simulink model "problem_6_case1"  (R2018a)
settings: Solver=ode1  StartTime=0.0  StopTime=4  FixedStep=0.0005  RelTol=1e-3
settings Model: Creator=chenxiaocong  LastModifiedBy=LvHonghao
settings CodeAppCC: StateflowObjectComments=on

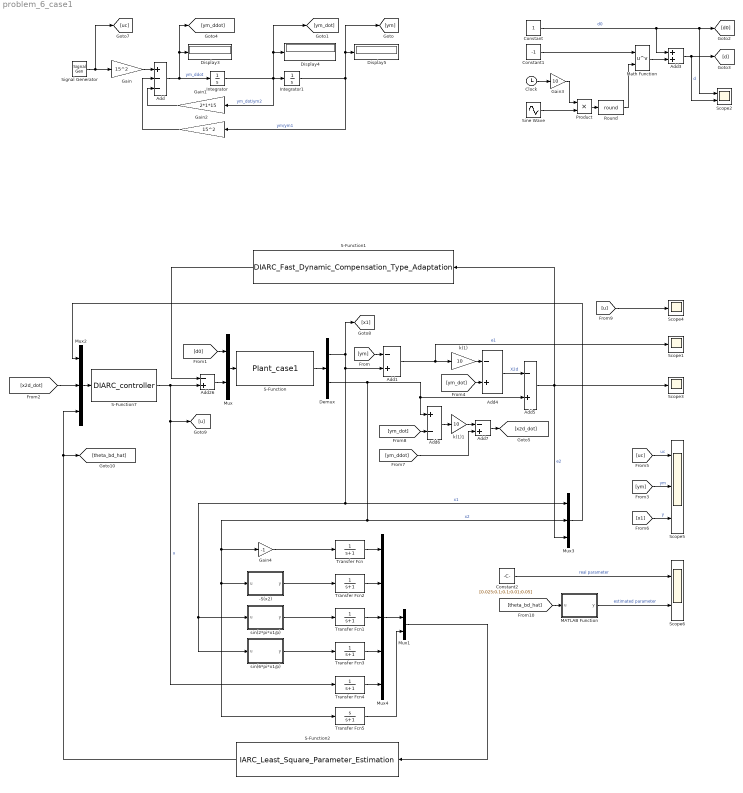
== system problem_6_case1 ==
  -S(x2) : MATLAB Function  TreatAsAtomicUnit=on
  Add : Sum  Inputs=+--
  Add{1,4..5,7,26} (5 alike) : Sum  Inputs=-+
  Add3 : Sum
  Add6 : Sum  Inputs=+-
  Clock : Clock
  Constant : Constant
  Constant1 : Constant  Value=-1
  Constant2 : Constant  Value=[0.025;0.1;0.1;0.01;0.05]
  Demux : Demux  Outputs=2
  Display3 : Display
  Display4 : Display
  Display5 : Display
  Gain : Gain  Gain=15^2
  Gain1 : Gain  Gain=2*1*15
  Gain2 : Gain  Gain=15^2
  Gain3 : Gain  Gain=10
  Gain4 : Gain  Gain=-1
  Integrator : Integrator
  Integrator1 : Integrator
  MATLAB Function : MATLAB Function  TreatAsAtomicUnit=on
  Math Function : Math  Operator=pow  SaturateOnIntegerOverflow=on
  Mux : Mux  Inputs=2
  Mux1 : Mux  Inputs=2
  Mux2 : Mux  Inputs=3
  Mux3 : Mux  Inputs=3
  Mux4 : Mux  Inputs=5
  Product : Product
  Round : Rounding  Operator=round
  S-Function : S-Function  FunctionName=Plant_case1  SFunctionDeploymentMode=off  EnableBusSupport=off
  S-Function1 : S-Function  FunctionName=DIARC_Fast_Dynamic_Compensation_Type_Adaptation  SFunctionDeploymentMode=off  EnableBusSupport=off
  S-Function2 : S-Function  FunctionName=IARC_Least_Square_Parameter_Estimation  SFunctionDeploymentMode=off  EnableBusSupport=off
  S-Function7 : S-Function  FunctionName=DIARC_controller  SFunctionDeploymentMode=off  EnableBusSupport=off
  Scope1 : Scope
  Scope2 : Scope  NumInputPorts=2
  Scope3 : Scope
  Scope4 : Scope
  Scope5 : Scope  NumInputPorts=3
  Scope6 : Scope  NumInputPorts=2
  Signal Generator : SignalGenerator  WaveForm=square  Amplitude=0.1  Frequency=1/1.2
  Sine Wave : Sin  Frequency=20  SampleTime=0
  Transfer Fcn{,1..4} (5 alike) : TransferFcn  Denominator=[1 1]
  Transfer Fcn5 : TransferFcn  Numerator=[1 0]  Denominator=[1 1]
  k(1) : Gain  Gain=10
  k(1)1 : Gain  Gain=10
  sin(2*pi*x1/p) : MATLAB Function  TreatAsAtomicUnit=on
  sin(6*pi*x1/p) : MATLAB Function  TreatAsAtomicUnit=on
  wires:
  Demux/2 -> Mux3/2, Transfer Fcn5/1, -S(x2)/1(u), Gain4/1, Add5/2, Add6/1  "x2"
  Add1/1 -> k(1)/1, Scope1/1  "e1"
  Gain2/1 -> Add/2
  Integrator1/1 -> Gain2/1, [ym], Display5/1  "ym/ym1"
  [ym_dot] -> Add6/2
  Add6/1 -> k(1)1/1
  [ym_dot] -> Add4/2
  Add4/1 -> Add5/1  "X2d"
  S-Function/1 -> Demux/1
  [d0] -> Mux/1
  Mux/1 -> S-Function/1
  Add3/1 -> [d], Scope2/2  "d"
  Constant/1 -> [d0], Scope2/1, Add3/1  "d0"
  k(1)/1 -> Add4/1
  k(1)1/1 -> Add7/1
  Add5/1 -> S-Function1/1, Mux3/3, Scope3/1  "e2"
  Integrator/1 -> Gain1/1, Integrator1/1, [ym_dot], Display4/1  "ym_dot/ym2"
  Gain1/1 -> Add/3
  Demux/1 -> Mux3/1, sin(6*pi*x1/p)/1(u), sin(2*pi*x1/p)/1(u), Add1/2, [x1]  "x1"
  Math Function/1 -> Add3/2
  Round/1 -> Math Function/2
  S-Function7/1 -> [u], Transfer Fcn4/1, Add26/2  "u"
  [ym] -> Add1/1
  Add/1 -> [ym_ddot], Display3/1, Integrator/1  "ym_ddot"
  [ym_ddot] -> Add7/2
  Gain/1 -> Add/1
  Add7/1 -> [x2d_dot]
  Constant1/1 -> Math Function/1
  Mux2/1 -> S-Function7/1
  [x2d_dot] -> Mux2/2
  [ym] -> Scope5/2  "ym"
  [uc] -> Scope5/1  "uc"
  [x1] -> Scope5/3  "y"
  [u] -> Scope4/1
  Constant2/1 -> Scope6/1  "real parameter"
  [theta_bd_hat] -> MATLAB Function/1(u)
  MATLAB Function/1(y) -> Scope6/2  "estimated parameter"
  S-Function2/1 -> Mux2/3, [theta_bd_hat]
  Mux3/1 -> Mux2/1
  Sine Wave/1 -> Product/2
  Clock/1 -> Gain3/1
  Product/1 -> Round/1
  Gain3/1 -> Product/1
  Signal Generator/1 -> [uc], Gain/1
  sin(6*pi*x1/p)/1(y) -> Transfer Fcn3/1
  sin(2*pi*x1/p)/1(y) -> Transfer Fcn1/1
  -S(x2)/1(y) -> Transfer Fcn2/1
  Transfer Fcn2/1 -> Mux4/2
  Mux4/1 -> Mux1/1
  Transfer Fcn4/1 -> Mux4/5
  Transfer Fcn/1 -> Mux4/1
  Gain4/1 -> Transfer Fcn/1
  Transfer Fcn1/1 -> Mux4/3
  Transfer Fcn5/1 -> Mux1/2
  Transfer Fcn3/1 -> Mux4/4
  Mux1/1 -> S-Function2/1
  Add26/1 -> Mux/2
  S-Function1/1 -> Add26/1

== matlab function problem_6_case1/MATLAB Function ==
  data: u input; y output
function y = fcn(u)
para_mid=[1;u(1:4)];
para_hat=para_mid/u(5);
y = para_hat;

== matlab function problem_6_case1/-S(x2) ==
  data: u input; y output
function y = fcn(u)
para=u*1000
if para>1
    y=1
elseif para<-1
    y=-1
else
    y=para;
end

== matlab function problem_6_case1/sin(2*pi*x1//p) ==
  data: u input; y output
function y = fcn(u)
p=0.06
y = sin(u*2*pi/p);

== matlab function problem_6_case1/sin(6*pi*x1//p) ==
  data: u input; y output
function y = fcn(u)

y = u;
